simulink model "FaultDectectionInPCB"  (R2020b)
settings: Solver=VariableStepAuto  StartTime=0.0  StopTime=100.0  RelTol=1e-3
undefined symbols (not defined in the file or in its folder): gray, none, Rec, SDTV, videoinput
libraries: visionstatistics x2, simulink x2, visiongeotforms x2, imaqlib x2, visionfilter x1, visionconversions x1, simulink_extras x1, visionanalysis x1, visionsources x1, dspstat3 x1
settings Model: Creator=Arif  LastModifiedBy=Arif

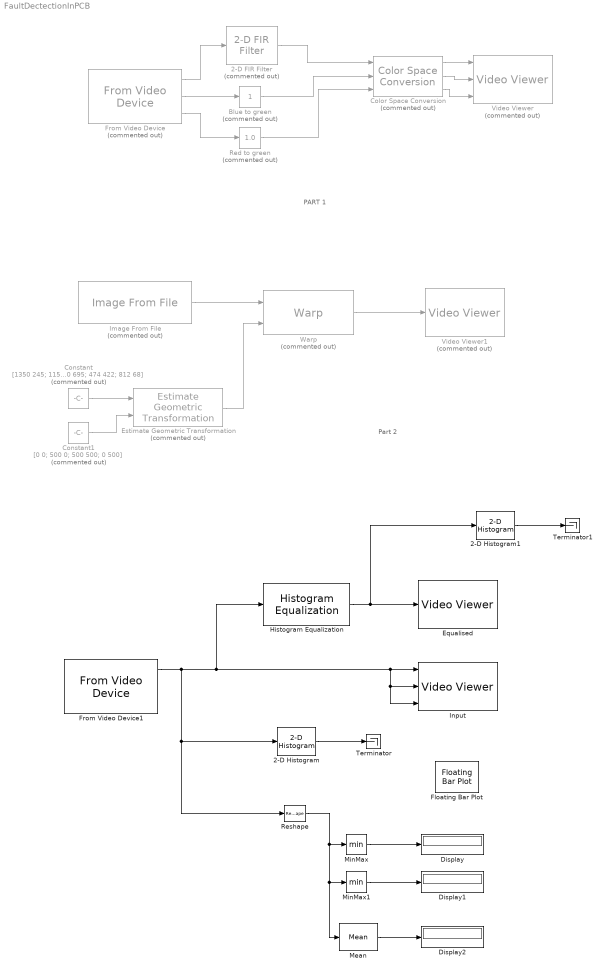
== system FaultDectectionInPCB ==
  note: Part 2
  note: PART 1
  2-D FIR Filter : visionfilter/2-D FIR Filter  Commented=on  separable=off  filtSrc=Specify via dialog  filterMtrx=[1/9 1/9 1/9; 1/9 1/9 1/9; 1/9 1/9 1/9]  verticalFilter=[4 0]  horizontalFilter=[4 0]  outSize=Same as input port I  padType=Constant  padSrc=Specify via dialog  padVal=0  method=Convolution  firstCoeffMode=Specify word length  firstCoeffWordLength=16  firstCoeffFracLength=14  firstCoeffSignedness=Signed  firstCoeffLastDataTypeStr=fixdt(1,16)  outputSignedness=Auto  accumLastDataTypeStr=Inherit: Same as product output  prodOutputMode=Binary point scaling  prodOutputWordLength=32  prodOutputFracLength=10  prodOutputLastDataTypeStr=fixdt([],32,10)  roundingMode=Floor  overflowMode=off  firstCoeffDataTypeStr=fixdt(1,16)  firstCoeffMin=[]  firstCoeffMax=[]  prodOutputDataTypeStr=fixdt([],32,10)  accumDataTypeStr=Inherit: Same as product output  outputMin=[]  outputMax=[]
      settings: SourceProductBaseCode=VP
  2-D Histogram : visionstatistics/2-D Histogram  umin=0  umax=1  nbins=256  operateOver=Entire input  normalized=off  run=off  reset=on  trigtype=None  Dimension=1  colComp=on  roundingMode=Floor  overflowMode=off
      settings: SourceProductBaseCode=VP
  2-D Histogram1 : visionstatistics/2-D Histogram  umin=0  umax=1  nbins=256  operateOver=Entire input  normalized=off  run=off  reset=on  trigtype=None  Dimension=1  colComp=on  roundingMode=Floor  overflowMode=off
      settings: SourceProductBaseCode=VP
  "Blue to green " : simulink/Math Operations/Slider Gain  Commented=on  gain=1  low=0  high=2
  Color Space Conversion : visionconversions/Color Space  Conversion  Commented=on  conversion=Obsolete  conversionActive=Y'CbCr to R'G'B'  wp_str=D65  rec=Rec. 601 (SDTV)  sys=1125/60/2:1  imagePorts=Separate color signals
  Constant : Constant  Commented=on  Value=[1350 245; 1150 695; 474 422; 812 68]
  Constant1 : Constant  Commented=on  Value=[0 0; 500 0; 500 500; 0 500]
  Display : Display
  Display1 : Display
  Display2 : Display
  Equalised : VideoViewer  FigPos=[2 517 957 409]
  Estimate Geometric Transformation : visiongeotforms/Estimate Geometric Transformation  Commented=on  tformType=Projective  isRandomSampling=on  algMethod=Random Sample Consensus (RANSAC)  distanceAlg=2.5  distanceGeo=2.5  numMethod=Specified value  sampleNum=500  desiredConfidence=99  maxSampleNum=1000  isStopSampling=off  percentStop=75  isRefineTForm=off  isReleaseMode=on  isOutputInlier=off  outDT4IntInput=Obsolete10a  outDT4IntInputActive=Single  isVarSizeAllowed=on
      settings: SourceProductBaseCode=VP
  Floating Bar Plot : simulink_extras/Additional Sinks/Floating Bar Plot  yLim=[0 200000]
      settings: SourceProductBaseCode=SL
  From Video Device : imaqlib/From Video Device  Commented=on  DeviceMenu=winvideo 1 (GENERAL WEBCAM)  Device=winvideo 1 (GENERAL WEBCAM)  ObjConstructor=videoinput('winvideo', 1)  VideoFormatMenu=MJPG_1280x720  VideoFormat=MJPG_1280x720  VideoSource=input1  ROIPosition=[0 0 720 1280]  EnableHWTrigger=off  TriggerConfiguration=none/none  SampleTime=1/30  OutputPortsMode=Separate color signals  DataType=single  CanDoHWTrigger=no  ReturnedColorSpace=YCbCr  BlockHandle=4.0002  ROIWidth=1280  ROIHeight=720  ROIColumn=0  ROIRow=0  EngXMLPath=D:\Arif\Programs\MATLAB_2020\toolbox\imaq\imaq\private  DevXMLPath=C:\ProgramData\MATLAB\SupportPackages\R2020b\toolbox\imaq\supportpackages\genericvideo\adaptor\win64  EngLibPath=D:\Arif\Programs\MATLAB_2020\toolbox\imaq\imaqblks\imaqmex\win64  ColorSpace=YCbCr  BayerSensorAlignment=grbg  ImaqMode=off
  From Video Device1 : imaqlib/From Video Device  DeviceMenu=(none)  Device=winvideo 1 (GENERAL WEBCAM)  ObjConstructor=videoinput('winvideo', 1)  VideoFormatMenu=(none)  VideoFormat=MJPG_1280x720  VideoSource=input1  ROIPosition=[0 0 720 1280]  EnableHWTrigger=off  TriggerConfiguration=none/none  SampleTime=1/30  OutputPortsMode=Separate color signals  DataType=single  CanDoHWTrigger=no  ReturnedColorSpace=YCbCr  BlockHandle=4.0002  ROIWidth=1280  ROIHeight=720  ROIColumn=0  ROIRow=0  EngXMLPath=D:\Arif\Programs\MATLAB_2020\toolbox\imaq\imaq\private  DevXMLPath=C:\ProgramData\MATLAB\SupportPackages\R2020b\toolbox\imaq\supportpackages\genericvideo\adaptor\win64  EngLibPath=D:\Arif\Programs\MATLAB_2020\toolbox\imaq\imaqblks\imaqmex\win64  ColorSpace=YCbCr  BayerSensorAlignment=grbg  ImaqMode=off
  Histogram Equalization : visionanalysis/Histogram Equalization  specify=Uniform  numbins=10  src=Specify via dialog  hist=ones(1,64)
      settings: SourceProductBaseCode=VP
  Image From File : visionsources/Image From File  Tag=vipblks_nd  Commented=on  FileName=D:\Arif\Documents\Meng units\DIP\myBoard.jpg  Ts=inf  imagePorts=One multidimensional signal  OutPortLabels=R|G|B  ImageDataType=Inherit from input image  sdImageDataType=uint(8)  Signed=on  WordLength=16  FractionLengthMode=User-defined  FractionLength=15
  Input : VideoViewer  imagePorts=separate color signals  FigPos=[2 1037 957 409]
  Mean : dspstat3/Mean  run=off  InputProcessing=Columns as channels (frame based)  reset_popup=None  directionMode=Each column  dimension=1  roiEnable=off  roiType=Rectangles  roiPortion=Entire ROI  roiOutput=Individual statistics for each ROI  roiFlag=off  roundingMode=Floor  overflowMode=off  outputDataTypeStr=Inherit: Same as accumulator  outputMin=[]  outputMax=[]  outputLastDataTypeStr=Inherit: Same as accumulator
  MinMax : MinMax
  MinMax1 : MinMax
  Red to green : simulink/Math Operations/Slider Gain  Commented=on  gain=1.0  low=0  high=2
  Reshape : Reshape
  Terminator : Terminator
  Terminator1 : Terminator
  Video Viewer : VideoViewer  Commented=on  imagePorts=separate color signals  FigPos=[2 1037 958 929]
  Video Viewer1 : VideoViewer  Commented=on  colormapValue=gray(256)  FigPos=[793 827 781 557]
  Warp : visiongeotforms/Warp  Commented=on  TransformMatrixSource=Input port  TransformMatrix=eye( 3 )  InterpolationMethod=Bilinear  BackgroundFillValue=0  OutputImagePositionSource=Same as input image  OutputImagePosition=[ 1, 1, 512, 512 ]  ROIInputPort=off  ROIValidityOutputPort=off  SimulateUsing=Interpreted execution
      settings: SourceProductBaseCode=VP
  wires:
  From Video Device/2 -> "Blue to green "/1
  From Video Device/3 -> Red to green/1
  "Blue to green "/1 -> Color Space Conversion/2
  Red to green/1 -> Color Space Conversion/3
  From Video Device/1 -> 2-D FIR Filter/1
  Color Space Conversion/1 -> Video Viewer/1
  Color Space Conversion/2 -> Video Viewer/2
  Color Space Conversion/3 -> Video Viewer/3
  2-D FIR Filter/1 -> Color Space Conversion/1
  Warp/1 -> Video Viewer1/1
  Estimate Geometric Transformation/1 -> Warp/2
  Image From File/1 -> Warp/1
  Constant/1 -> Estimate Geometric Transformation/1
  Constant1/1 -> Estimate Geometric Transformation/2
  From Video Device1/1 -> Histogram Equalization/1, Input/3, Input/2, Input/1, Reshape/1, 2-D Histogram/1
  2-D Histogram/1 -> Terminator/1
  Reshape/1 -> Mean/1, MinMax1/1, MinMax/1
  MinMax/1 -> Display/1
  MinMax1/1 -> Display1/1
  Mean/1 -> Display2/1
  Histogram Equalization/1 -> 2-D Histogram1/1, Equalised/1
  2-D Histogram1/1 -> Terminator1/1
